simulink model "modelo4"  (R2019a)
settings: Solver=FixedStepAuto  StartTime=0.0  StopTime=tfinal  FixedStep=0.0001  RelTol=1e-3
values from neighbouring files (symbols this model uses):
  A = 4*10^(-4)    (= 0.0004)    [nonlinear.m]    (also in sim2.m = [zeros(2) eye(2);Ke*eye(2) -Ge]; sim3.m = [zeros(2) eye(2);Ke*eye(2) -Ge]; sim4.m = [zeros(2) eye(2);Ke*eye(2) -Ge])
  A_hat = Auu - Lr*Aau    [sim3.m]    (also in sim4.m)
  B = (1/J)*d*b*ki*[zeros(2);eye(2)]    [sim2.m]    (also in sim3.m = (1/J)*d*b*gi*[zeros(2);eye(2)]; sim4.m = (1/J)*d*b*gi*[zeros(2);eye(2)])
  B_hat = A_hat*Lr + Aua -Lr*Aaa    [sim3.m]    (also in sim4.m)
  C = [eye(2) zeros(2)]    [sim2.m]    (also in sim3.m; sim4.m)
  C_hat = [zeros(2);eye(2)]    [sim3.m]    (also in sim4.m)
  D = zeros(2)    [sim2.m]    (also in sim3.m = zeros(4,2); sim4.m = zeros(4,2))
  D_hat = [eye(2);Lr]    [sim3.m]    (also in sim4.m)
  F = lqr(A,B,Q,R)    [descentralizado.m]    (also in sim2.m = Fdn)
  G = Bu - Lr*Ba    [sim3.m]    (also in sim4.m)
  L = place(A',C',5*e).'    [sim3.m]    (also in sim4.m)
  omega = 4000    [sim2.m]    (also in sim3.m = 356; sim4.m = 3204)
  x0 = [0.0002;-0.0002;0;0]    [sim2.m]    (also in sim3.m; sim4.m)
settings Model: Creator=vinic  LastModifiedBy=vinic
settings DataIOCC: ReturnWorkspaceOutputs=off
settings DebuggingCC: PregeneratedLibrarySubsystemCodeDiagnostic=none  ArithmeticOperatorsInVariantConditions=warning
settings SFSimCC: SimUseLocalCustomCode=off
settings RTWCC: RTWUseLocalCustomCode=off

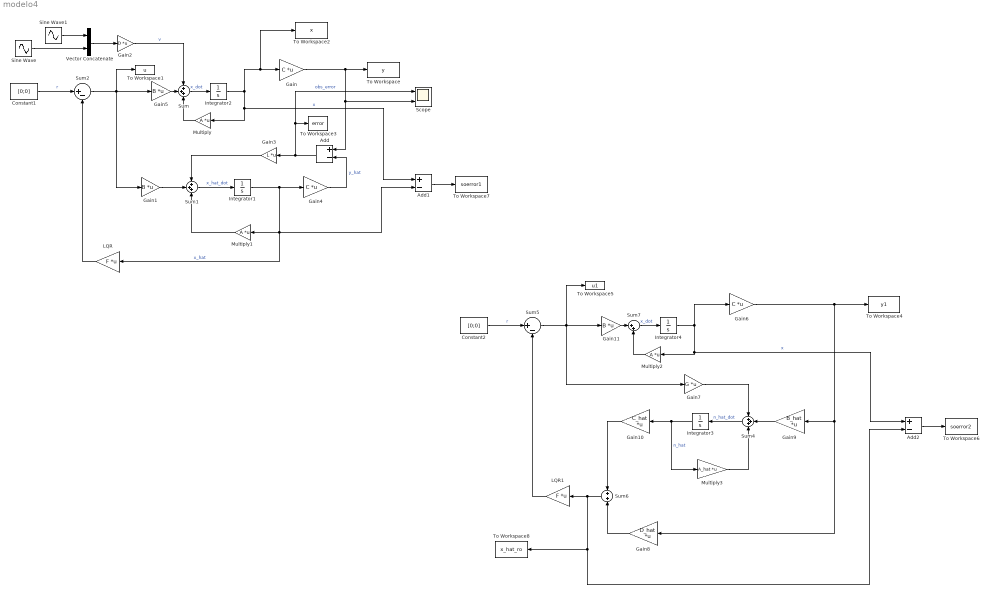
== system modelo4 ==
  Add : Sum  Inputs=+-
  Add1 : Sum  Inputs=+-
  Add2 : Sum  Inputs=+-
  Constant1 : Constant  Value=[0;0]  VectorParams1D=off
  Constant2 : Constant  Value=[0;0]  VectorParams1D=off
  Gain : Gain  Gain=C  Multiplication=Matrix(K*u)
  Gain1 : Gain  Gain=B  Multiplication=Matrix(K*u)
  Gain10 : Gain  Gain=C_hat  Multiplication=Matrix(K*u)
  Gain11 : Gain  Gain=B  Multiplication=Matrix(K*u)
  Gain2 : Gain  Gain=D  Multiplication=Matrix(K*u)
  Gain3 : Gain  Gain=L  Multiplication=Matrix(K*u)
  Gain4 : Gain  Gain=C  Multiplication=Matrix(K*u)
  Gain5 : Gain  Gain=B  Multiplication=Matrix(K*u)
  Gain6 : Gain  Gain=C  Multiplication=Matrix(K*u)
  Gain7 : Gain  Gain=G  Multiplication=Matrix(K*u)
  Gain8 : Gain  Gain=D_hat  Multiplication=Matrix(K*u)
  Gain9 : Gain  Gain=B_hat  Multiplication=Matrix(K*u)
  Integrator1 : Integrator  InitialCondition=[0;0;0;0]
  Integrator2 : Integrator  InitialCondition=x0
  Integrator3 : Integrator  InitialCondition=[0;0]
  Integrator4 : Integrator  InitialCondition=x0
  LQR : Gain  Gain=F  Multiplication=Matrix(K*u)
  LQR1 : Gain  Gain=F  Multiplication=Matrix(K*u)
  Multiply : Gain  Gain=A  Multiplication=Matrix(K*u)
  Multiply1 : Gain  Gain=A  Multiplication=Matrix(K*u)
  Multiply2 : Gain  Gain=A  Multiplication=Matrix(K*u)
  Multiply3 : Gain  Gain=A_hat  Multiplication=Matrix(K*u)
  Scope : Scope  NumInputPorts=2
  Sine Wave : Sin  Amplitude=-1  Frequency=omega  SampleTime=0
  Sine Wave1 : Sin  Frequency=omega  Phase=-pi/2  SampleTime=0
  Sum : Sum  Inputs=+++
  Sum1 : Sum  Inputs=+++
  Sum2 : Sum  Inputs=|+-
  Sum4 : Sum  Inputs=+++
  Sum5 : Sum  Inputs=|+-
  Sum6 : Sum
  Sum7 : Sum  Inputs=|++
  To Workspace : ToWorkspace  VariableName=y  SampleTime=-1
  To Workspace1 : ToWorkspace  VariableName=u  SampleTime=-1
  To Workspace2 : ToWorkspace  VariableName=x  SampleTime=-1
  To Workspace3 : ToWorkspace  VariableName=error  SaveFormat=Timeseries  SampleTime=-1
  To Workspace4 : ToWorkspace  VariableName=y1  SampleTime=-1
  To Workspace5 : ToWorkspace  VariableName=u1  SampleTime=-1
  To Workspace6 : ToWorkspace  VariableName=soerror2  SampleTime=-1
  To Workspace7 : ToWorkspace  VariableName=soerror1  SampleTime=-1
  To Workspace8 : ToWorkspace  VariableName=x_hat_ro  SampleTime=-1
  Vector Concatenate : Concatenate
  wires:
  Sum2/1 -> Gain1/1, To Workspace1/1, Gain5/1
  Integrator2/1 -> Add1/1, Multiply/1, To Workspace2/1, Gain/1  "x"
  Gain/1 -> Add/1, Scope/2, To Workspace/1
  Gain5/1 -> Sum/2
  Multiply/1 -> Sum/3
  Sum/1 -> Integrator2/1  "x_dot"
  Gain2/1 -> Sum/1  "v"
  LQR/1 -> Sum2/2
  Sine Wave1/1 -> Vector Concatenate/1
  Sine Wave/1 -> Vector Concatenate/2
  Vector Concatenate/1 -> Gain2/1
  Constant1/1 -> Sum2/1  "r"
  Integrator1/1 -> Gain4/1, Add1/2, LQR/1, Multiply1/1  "x_hat"
  Sum1/1 -> Integrator1/1  "x_hat_dot"
  Gain1/1 -> Sum1/2
  Multiply1/1 -> Sum1/3
  Gain4/1 -> Add/2  "y_hat"
  Add/1 -> Gain3/1, Scope/1, To Workspace3/1  "obs_error"
  Gain3/1 -> Sum1/1
  Multiply2/1 -> Sum7/2
  Constant2/1 -> Sum5/1  "r"
  Sum7/1 -> Integrator4/1  "x_dot"
  Gain6/1 -> Gain8/1, Gain9/1, To Workspace4/1
  Sum5/1 -> Gain7/1, To Workspace5/1, Gain11/1
  Integrator4/1 -> Add2/1, Multiply2/1, Gain6/1  "x"
  Multiply3/1 -> Sum4/3
  Integrator3/1 -> Gain10/1, Multiply3/1  "n_hat"
  LQR1/1 -> Sum5/2
  Gain11/1 -> Sum7/1
  Sum4/1 -> Integrator3/1  "n_hat_dot"
  Gain7/1 -> Sum4/1
  Gain9/1 -> Sum4/2
  Gain10/1 -> Sum6/1
  Gain8/1 -> Sum6/2
  Sum6/1 -> To Workspace8/1, Add2/2, LQR1/1
  Add1/1 -> To Workspace7/1
  Add2/1 -> To Workspace6/1
